simulink model "planner_contral"  (R2023b)
settings: Solver=FixedStepAuto  StartTime=0  StopTime=inf  FixedStep=0.001  RelTol=1e-3
undefined symbols (not defined in the file): aubr, c_factor, cf, cr, iniObsHeading1, iniObsHeading2, iniObsPos1, iniObsPos2, KD_PID_distance, KD_PID_speed, KI_PID_distance, KI_PID_speed, KP_PID_distance, KP_PID_speed, la, lb, LQR_K1, LQR_K2, LQR_K3, LQR_K4, m, rack_displacement, refInfo_obs1, refInfo_obs2, right_wheel_ground, rightWaypoints, tablebr, vubr, vx_break_point
libraries: Solver_SF x1
(part 5 of 8)

== matlab function planner_contral/decision_planning/EMplanner/generate convex space_base ==
  data: dp_speed_s input; s_lb output; dp_speed_t input; path_index2s input; static_obs_s_lb input; static_obs_s_ub input; static_obs_t_lb input; static_obs_t_ub input; dynamic_obs_s_lb input; dynamic_obs_s_ub input; dynaimc_obs_t_lb input; dynaimc_obs_t_ub input; s_ub output; s_dot_lb output; s_dot_ub output; trajectory_kappa_init input; max_lateral_accel input; static_s_ub output; static_s_lb output
function [s_lb,s_ub,s_dot_lb,s_dot_ub, static_s_ub,static_s_lb] = fcn(dp_speed_s,dp_speed_t,path_index2s,static_obs_s_lb,static_obs_s_ub,static_obs_t_lb,static_obs_t_ub,...
   dynamic_obs_s_lb,dynamic_obs_s_ub,dynaimc_obs_t_lb,dynaimc_obs_t_ub,trajectory_kappa_init,max_lateral_accel)
%generate convex space_base 该函数将计算出s,s_dot的上下界，开辟凸空间供二次规划使用
% dp_speed_s t 最多有16个，输出初始化n = 16
n = 16;
static_s_lb = ones(n,1)*-inf;
static_s_ub = ones(n,1)*inf;
dynamic_s_lb = ones(n,1)*-inf;
dynamic_s_ub = ones(n,1)*inf;
s_lb=ones(n,1)*-inf;
s_ub=ones(n,1)*inf;
s_dot_lb = ones(n,1)*-inf;
s_dot_ub = ones(n,1)*inf;
path_index2s_end_index = length(path_index2s);
dp_speed_end_index = length(dp_speed_s);

% path_index2s也是有缓冲的，找到有效的path_index2s的末尾的位置，赋值给path_index2s_end_index
for k = 2:length(path_index2s)
    if path_index2s(k) == 0 && path_index2s(k-1) ~= 0
        path_index2s_end_index = k - 1;
        break;
    end
    path_index2s_end_index = k;
end
% 找到dp_speed_s中有效的位置，赋值给dp_speed_end_index
for k = 1:length(dp_speed_s)
    if isnan(dp_speed_s(k))
        dp_speed_end_index = k - 1;
        break;
    end
end

for i = 1:n
    % 该循环将施加车辆动力学约束
    if isnan(dp_speed_s(i))
        break;
    end
    cur_s = dp_speed_s(i);
    % 通过插值的方式找到cur_s 所对应的曲率
    cur_kappa = interp1(path_index2s(1:path_index2s_end_index),trajectory_kappa_init(1:path_index2s_end_index),cur_s);
    % a = v^2 * k => v^2 = a/k 注意除0保护
    max_speed =  sqrt(max_lateral_accel / (abs(cur_kappa) + 1e-10));
    min_speed = 0;
    s_dot_lb(i) = min_speed;
    s_dot_ub(i) = max_speed;    
end



for i = 1:length(static_obs_s_lb)
    if isinf(static_obs_s_lb(i))
        continue;
    end
    % 取s t 直线的中点，作为obs_s obs_t 的坐标 
    static_obs_t = (static_obs_t_lb(i) + static_obs_t_ub(i)) / 2;
    static_obs_s = (static_obs_s_lb(i) + static_obs_s_ub(i)) / 2;
    % 插值找到当t = obs_t时，dp_speed_s 的值
    dp_s = interp1([0;dp_speed_t(1:dp_speed_end_index)],[0;dp_speed_s(1:dp_speed_end_index)],static_obs_t );
    if isnan(dp_s)
        continue;
    end
    [letf_index,right_index]=getTBoundindex(static_obs_t,dp_speed_t,dp_speed_end_index);
    if letf_index==0
        continue
    end
    if static_obs_s > dp_s
        % 决策为减速避让
        for m = letf_index:right_index
            % 在t_lb_index:t_ub_index的区间上 s的上界不可以超过障碍物st斜直线
            static_s_ub(m) = min(static_s_ub(m),static_obs_s_lb(i) -1.2);
        end
    else 
        % 决策为加速超车
        for  m = letf_index:right_index
             % 在t_lb_index:t_ub_index的区间上 s的下界不能小于障碍物st斜直线
            static_s_lb(m) = max(static_s_lb(m),static_obs_s_ub(i)+1.2 );
        end
    end

end
  
%计算动态障碍物上下凸空间边界
for i = 1:length(dynamic_obs_s_lb)
    if  isinf(dynamic_obs_s_lb(i))
        continue;
    end
    % 取s t 直线的中点，作为obs_s obs_t 的坐标 
    dynamic_obs_t = (dynaimc_obs_t_lb(i) + dynaimc_obs_t_ub(i)) / 2;
    dynamic_obs_s = (dynamic_obs_s_lb(i) + dynamic_obs_s_ub(i)) / 2;
    % 插值找到当t = obs_t时，dp_speed_s 的值
    dp_s = interp1([0;dp_speed_t(1:dp_speed_end_index)],[0;dp_speed_s(1:dp_speed_end_index)],dynamic_obs_t);
    if isnan(dp_s)
        continue;
    end
    [letf_index,right_index]=getTBoundindex(dynamic_obs_t,dp_speed_t,dp_speed_end_index);
    if letf_index==0
        continue
    end
    if dynamic_obs_s> dp_s
        % 决策为减速避让
        for m = letf_index:right_index
            % 在t_lb_index:t_ub_index的区间上 s的上界不可以超过障碍物st斜直线
            dynamic_s_ub(m) = min(dynamic_s_ub(m),dynamic_obs_s_lb(i) -1.2);
        end
    else 
        % 决策为加速超车
        for  m = letf_index:right_index
             % 在t_lb_index:t_ub_index的区间上 s的下界不能小于障碍物st斜直线
            dynamic_s_lb(m) = max(dynamic_s_lb(m) +1.2,dynamic_obs_s_ub(i));
        end
    end

end
%开始做决策，判断凸空间
 for k=1:n
     if isnan(dp_speed_s(k))
        break;
     end
     %该点没有动态障碍物点以及静态障碍物点
     if  isinf(static_s_lb(k))&& isinf(dynamic_s_lb(k))&&isinf(static_s_ub(k))&& isinf(dynamic_s_ub(k))
         continue
     end
     %针对曲线在静态障碍物上方
     if ~isinf(static_s_lb(k))&& isinf(dynamic_s_lb(k))&&isinf(static_s_ub(k))&& isinf(dynamic_s_ub(k))
         s_lb(k)=static_s_lb(k);
         s_ub(k)=static_s_ub(k);
       
     end
     %曲线在静态障碍物下方
     if isinf(static_s_lb(k))&& isinf(dynamic_s_lb(k))&&~isinf(static_s_ub(k))&& isinf(dynamic_s_ub(k))
         s_lb(k)=static_s_lb(k);
         s_ub(k)=static_s_ub(k);
        
     end
     %曲线在动态障碍物上方
     if isinf(static_s_lb(k))&& ~isinf(dynamic_s_lb(k))&&isinf(static_s_ub(k))&& isinf(dynamic_s_ub(k))
         s_lb(k)=dynamic_s_lb(k);
         s_ub(k)=dynamic_s_ub(k);
       
     end
     %曲线在动态障碍物下方
     if isinf(static_s_lb(k))&& isinf(dynamic_s_lb(k))&&isinf(static_s_ub(k))&& ~isinf(dynamic_s_ub(k))
         s_lb(k)=dynamic_s_lb(k);
         s_ub(k)=dynamic_s_ub(k);
        
     end
     %
     if ~isnan(static_s_ub(k))&&~isnan(dynamic_s_lb(k))
         s_lb(k)=dynamic_s_lb(k);
         s_ub(k)=static_s_ub(k);
     end
     if ~isnan(static_s_lb(k))&&~isnan(dynamic_s_ub(k))
         s_lb(k)=static_s_lb(k);
         s_ub(k)=dynamic_s_ub(k);
     end
     %
     if ~isnan(static_s_ub(k))&&~isnan(dynamic_s_ub(k))
          if dynamic_s_ub(k)>static_s_ub(k)
            s_ub(k)=static_s_ub(k);
          else
            s_ub(k)=dynamic_s_ub(k);
          end
     end
     %
     if ~isnan(static_s_lb(k))&&~isnan(dynamic_s_lb(k))
          if dynamic_s_lb(k)>static_s_lb(k)
            s_lb(k)=dynamic_s_lb(k);
          else
            s_lb(k)=static_s_lb(k);
          end
     end




end

end     

%该函数是为了获取当前t所对应的轨迹索引
function [left,right]=getTBoundindex(obs_t,dp_speed_t_,dp_speed_end_index_)
  %初始化参数
  left=0;
  right=0;
  %遍历dp_speed_t,找到当前obs_t_lb,obs_t_ub处于dp_speed_t的位置范围

  %判断索引位置
  for j=1:length(dp_speed_t_)
      %获取障碍物的t索引范围
      if dp_speed_t_(1)>obs_t           %说明障碍物当前时刻没有对应的索引值
          break;
      end
      if dp_speed_t_(j)< obs_t && dp_speed_t_(j + 1) > obs_t
          left=max(1,j);
          right=min(j+1,dp_speed_end_index_);
          break; 
      end
      if dp_speed_t_(j)== obs_t
          left=max(1,j);
          right=min(j,dp_speed_end_index_);
      end

  end

end

== matlab function planner_contral/decision_planning/EMplanner/obs/1 ==
  data: dynamic_obs_x_set_gcs input; dynamic_obs_y_set_gcs input; dynamic_obs_heading_set_gcs input; dynamic_obs_velocity_set_gcs input; dynamic_obs1_x_pre output; dynamic_obs1_y_pre output; dynamic_obs1_vx_set output; dynamic_obs1_vy_set output; pre_obs1 input
function [dynamic_obs1_x_pre,dynamic_obs1_y_pre,dynamic_obs1_vx_set,dynamic_obs1_vy_set ]...
    = fcn(dynamic_obs_x_set_gcs,dynamic_obs_y_set_gcs,dynamic_obs_heading_set_gcs,dynamic_obs_velocity_set_gcs,pre_obs1)

%该函数将分类静态障碍物和动态障碍物
%输出初始化
n = 32;

dynamic_obs1_x_pre = ones(n,1)*nan;
dynamic_obs1_y_pre = ones(n,1)*nan;
dynamic_obs1_vx_set = ones(n,1)*nan;
dynamic_obs1_vy_set = ones(n,1)*nan;
dynamic_obs1_heading_set = ones(n,1)*nan;
% dynamic_obs2_x_pre = ones(n,1)*nan;
% dynamic_obs2_y_pre = ones(n,1)*nan;
% dynamic_obs2_vx_set = ones(n,1)*nan;
% dynamic_obs2_vy_set = ones(n,1)*nan;
pre_tra_obs1_x=pre_obs1(:,1)';
pre_tra_obs1_y=pre_obs1(:,2)';
% pre_tra_obs2_x=pre_obs1(:,1)';
% pre_tra_obs2_y=pre_obs1(:,2)';
count_dynamic = 1;
for i = 1:length(dynamic_obs_x_set_gcs)
    if ~isnan(dynamic_obs_x_set_gcs(i))
        if i==1
        dynamic_obs1_x_pre(1) = dynamic_obs_x_set_gcs(i);
        dynamic_obs1_y_pre(1) =dynamic_obs_y_set_gcs(i);
            dynamic_obs1_vx_set(1) =dynamic_obs_velocity_set_gcs(i)*cos(dynamic_obs_heading_set_gcs(i));
            dynamic_obs1_vy_set(1) = dynamic_obs_velocity_set_gcs(i)*sin(dynamic_obs_heading_set_gcs(i));

         for j=1:length(pre_tra_obs1_x(1,:))
              %交换位置
            dynamic_obs1_x_pre(j+1) =pre_tra_obs1_x(1,j);
            dynamic_obs1_y_pre(j+1) =pre_tra_obs1_y(1,j);
            dynamic_obs1_vx_set(j+1) =dynamic_obs_velocity_set_gcs(i)*cos(dynamic_obs_heading_set_gcs(i));
            dynamic_obs1_vy_set(j+1) = dynamic_obs_velocity_set_gcs(i)*sin(dynamic_obs_heading_set_gcs(i));

         end
      for z=1:length(dynamic_obs1_x_pre)-1
          if dynamic_obs1_x_pre(z+1)<dynamic_obs1_x_pre(z)
              temp_x=dynamic_obs1_x_pre(z+1);
              temp_y=dynamic_obs1_y_pre(z+1);
              dynamic_obs1_x_pre(z+1)=dynamic_obs1_x_pre(z);
              dynamic_obs1_y_pre(z+1)=dynamic_obs1_y_pre(z);
              dynamic_obs1_x_pre(z)=temp_x;
              dynamic_obs1_y_pre(z)=temp_y;
          else
              break
          end
      end
 
 

      end



        %在此处增密路径变为80个点
         

           %计算动态障碍物航向角
%           [path_heading_,path_kappa_] = fcn(path_x,path_y)


        end

%         if i==2
%         dynamic_obs2_x_pre(1) = obs_x_set_gcs(i);
%         dynamic_obs2_y_pre(1) = obs_y_set_gcs(i);
%         for j=1:length(pre_tra_obs2_x(1,:))
%             dynamic_obs2_x_pre(j+1) =pre_tra_obs2_x(1,j);
%             dynamic_obs2_y_pre(j+1) =pre_tra_obs2_y(1,j);
% 
%         end 
%             dynamic_obs2_vx_set(1) = obs_velocity_set_gcs(i)*cos(obs_heading_set_gcs(i));
%             dynamic_obs2_vy_set(1) = obs_velocity_set_gcs(i)*sin(obs_heading_set_gcs(i));
%         end
%             
      count_dynamic = count_dynamic + 1;    
     end
% end

% function[tra_x,tra_y]=Den(tra_x_init,tra_y_init)
% %定义增密数组长度
% n=80;
% tra_x=ones(n,1);
% tra_y=ones(n,1);
% 
% 
% 
% 
% end
% 
% 
% 
% 
% function [path_heading,path_kappa] = fcn(path_x,path_y)
% %该函数将计算path的切线方向与x轴的夹角和曲率
% %输入：path_x,y路径坐标
% %输出：path heading kappa 路径的heading和曲率
% %原理 heading = arctan(dy/dx);
% %     kappa = dheading/ds;
% %     ds = (dx^2 + dy^2)^0.5
% 
% %注意，角度的多值性会带来很大的麻烦，需要慎重处理
% %例，x 与 x + 2pi往往代表同一个角度，这种多值性在计算曲率会带来麻烦
% %比如 原本是(0.1 - (-0.1))/ds，但如果计算出的-0.1多了一个2pi
% %kappa就等于(0.1 - (-0.1 + 2*pi))/ds，曲率会变得非常大
% %还有若采用中点欧拉法计算heading时，(即使用(y2 - y1)/(x2 - x1)的反正切计算一个角度 ，用(y1 - y0)/(x1
% %-x0)的反正切又计算一个角度，然后加起来除以2),如果精确值是 (a1 + a2)/2,但最终计算的结果可能是(a1 + a2 + 2pi)/2
% % 还有 tan(x) = tan(x + pi) 所以arctan(tan(x))可能等于x，也可能等于x + pi
% % 角度的处理非常麻烦，而且角度处理不当往往是许多奇怪错误的源头
% 
% dx = diff(path_x);
% dy = diff(path_y);
% %用中点欧拉法要比向前欧拉法向后欧拉法更精确，但是也可能计算出的结果比精确值多一个pi
% %在这里对dx,dy做中点欧拉法，使用四象限反正切计算角度
% dx_pre = [dx(1);dx];
% dx_after = [dx;dx(end)];
% dx_final = (dx_pre + dx_after)/2;
% 
% dy_pre = [dy(1);dy];
% dy_after = [dy;dy(end)];
% dy_final = (dy_pre + dy_after)/2;
% 
% ds_final = sqrt(dx_final.^2 + dy_final.^2);
% path_heading = atan2(dy_final,dx_final);
% 
% dheading = diff(path_heading);
% dheading_pre = [dheading(1);dheading];
% dheading_after = [dheading;dheading(end)];
% dheading_final = (dheading_pre + dheading_after) / 2;
% %为了防止dheading出现多一个2pi的错误，假设真实的dheading较小，用sin(dheading)近似dheading
% path_kappa = sin(dheading_final) ./ ds_final;
% end

== matlab function planner_contral/decision_planning/EMplanner/spee planning with quadratic programming (qp)_base ==
  data: plan_start_s_dot input; qp_s_init output; plan_start_s_dot2 input; dp_speed_s input; dp_speed_t input; s_lb input; s_ub input; s_dot_lb input; s_dot_ub input; qp_s_dot_init output; qp_s_dot2_init output; relative_time_init output; w_cost_s_dot2 input; w_cost_v_ref input; w_cost_jerk input; w_ref_s input; speed_reference input
function [qp_s_init,qp_s_dot_init,qp_s_dot2_init,relative_time_init] = fcn(plan_start_s_dot,...
    plan_start_s_dot2,dp_speed_s,dp_speed_t,s_lb,s_ub,s_dot_lb,s_dot_ub,w_cost_s_dot2,w_cost_v_ref,w_cost_jerk,w_ref_s,speed_reference)
%速度二次规划
% 输入：规划起点plan_start_s_dot,plan_start_s_dot2
%       动态规划结果dp_speed_s,dp_speed_t
%       凸空间约束 s_lb,s_ub,s_dot_lb,s_dot_ub
%       加速度代价权重，推荐速度代价权重，jerk代价权重w_cost_s_dot2,w_cost_v_ref,w_cost_jerk
%       参考速度speed_reference
% 输出：速度曲线qp_s_init,qp_s_dot_init,qp_s_dot2_init,relative_time_init
coder.extrinsic("quadprog")
% 由于dp的结果未必是16，该算法将计算dp_speed_end到底是多少
dp_speed_end = 16;
for i = 1:length(dp_speed_s)
    
    if isnan(dp_speed_s(i))
        dp_speed_end = i - 1;
        break;
    end
end
% 由于dp_speed_end实际上是不确定的，但是输出要求必须是确定长度的值，因此
% 输出初始化选择dp_speed_end的最大值 + 规划起点作为输出初始化的规模
n = 17;

qp_s_init = ones(n,1) * nan;
qp_s_dot_init = ones(n,1) * nan;
qp_s_dot2_init = ones(n,1) * nan;
relative_time_init = ones(n,1) * nan;
s_end = dp_speed_s(dp_speed_end);
% 此时dp_speed_end表示真正有效的dp_speed_t的元素个数，取出dp_speed_t有效的最后一个元素作为规划的时间终点
% 记为recommend_T
recommend_T = dp_speed_t(dp_speed_end);
% qp的规模应该是dp的有效元素的个数 + 规划起点
qp_size = dp_speed_end + 1;
% 连续性约束矩阵初始化，这里的等式约束应该是 Aeq'*X == beq 有转置
Aeq = zeros(3*qp_size,2*qp_size - 2);
beq = zeros(2*qp_size - 2,1);
% 不等式约束初始化
lb = ones(3*qp_size,1);
ub = lb;
% 计算采样间隔时间dt,连续性约束
dt = recommend_T/dp_speed_end;
A_sub =[1,0;
        dt,1;
        (1/3)*dt^2,(1/2)*dt;
        -1,0;
        0,-1;
        (1/6)*dt^2,dt/2];
for i = 1:qp_size - 1
    Aeq(3*i-2:3*i+3,2*i-1:2*i) = A_sub;
end
% 这里初始化不允许倒车约束，也就是 s(i) - s(i+1) <= 0
A = zeros(qp_size-1,3*qp_size);
b = zeros(qp_size-1,1);
for i = 1:qp_size-1
    A(i,3*i - 2) = 1;
    A(i,3*i + 1) = -1;
end
% 由于生成的凸空间约束s_lb s_ub不带起点，所以lb(i) = s_lb(i-1) 以此类推
% 允许最小加速度为-6 最大加速度为4(基于车辆动力学)
for i = 2:qp_size
   lb(3*i - 2) = s_lb(i-1);
   lb(3*i - 1) = s_dot_lb(i-1);
   lb(3*i) = -6;
   ub(3*i - 2) = s_ub(i-1);
   ub(3*i - 1) = s_dot_ub(i-1);
   ub(3*i) = 4;
end
% 起点约束
lb(1) = 0;
lb(2) = plan_start_s_dot;
lb(3) = plan_start_s_dot2;
ub(1) = lb(1);
ub(2) = lb(2);
ub(3) = lb(3);
% 加速度代价 jerk代价 以及推荐速度代价
A_s_dot2 = zeros(3*qp_size,3*qp_size);
A_jerk = zeros(3*qp_size,qp_size - 1);
A_ref = zeros(3*qp_size,3*qp_size);
A_ref_s = zeros(3*qp_size,3*qp_size);
A4_sub =[0;0;1;0;0;-1];
for i = 1:qp_size
    A_s_dot2(3*i,3*i) = 1;
    A_ref(3*i-1,3*i-1) = 1;
    A_ref_s(3*i-2,3*i-2)=1;
end
for i = 1:qp_size - 1   
   A_jerk(3*i-2:3*i+3,i:i) = A4_sub;
end
% 生成H f
H = w_cost_s_dot2 * (A_s_dot2 * A_s_dot2') + w_cost_jerk * (A_jerk * A_jerk') + w_cost_v_ref * (A_ref * A_ref')+w_ref_s*(A_ref_s * A_ref_s');
H = 2*H;
f = zeros(3*qp_size,1);
for i = 1:qp_size
    f(3*i-1) =  - 2 * w_cost_v_ref * speed_reference;  %这里应该晖多加一个代价
   
end
for i=1:dp_speed_end
      f(3*i-2) =  - 2 * w_ref_s * dp_speed_s(i);  %这里应该晖多加一个代价
end

% 计算二次规划
X = quadprog(H,f,A,b,Aeq',beq,lb,ub);
% 将结果输出
for i = 1:qp_size
   qp_s_init(i) = X(3*i - 2);
   qp_s_dot_init(i) = X(3*i - 1);
   qp_s_dot2_init(i) = X(3*i);
   relative_time_init(i) = (i - 1)*dt;
end

== matlab function planner_contral/decision_planning/EMplanner/spee planning with quadratic programming (qp)_1 ==
  data: plan_start_s_dot input; qp_s_init output; plan_start_s_dot2 input; dp_speed_s input; dp_speed_t input; s_lb input; s_ub input; s_dot_lb input; s_dot_ub input; qp_s_dot_init output; qp_s_dot2_init output; relative_time_init output; w_cost_s_dot2 input; w_cost_v_ref input; w_cost_jerk input; w_ref_s input; speed_reference input
function [qp_s_init,qp_s_dot_init,qp_s_dot2_init,relative_time_init] = fcn(plan_start_s_dot,...
    plan_start_s_dot2,dp_speed_s,dp_speed_t,s_lb,s_ub,s_dot_lb,s_dot_ub,w_cost_s_dot2,w_cost_v_ref,w_cost_jerk,w_ref_s,speed_reference)
%速度二次规划
% 输入：规划起点plan_start_s_dot,plan_start_s_dot2
%       动态规划结果dp_speed_s,dp_speed_t
%       凸空间约束 s_lb,s_ub,s_dot_lb,s_dot_ub
%       加速度代价权重，推荐速度代价权重，jerk代价权重w_cost_s_dot2,w_cost_v_ref,w_cost_jerk
%       参考速度speed_reference
% 输出：速度曲线qp_s_init,qp_s_dot_init,qp_s_dot2_init,relative_time_init
coder.extrinsic("quadprog")
% 由于dp的结果未必是16，该算法将计算dp_speed_end到底是多少
dp_speed_end = 16;
for i = 1:length(dp_speed_s)
    
    if isnan(dp_speed_s(i))
        dp_speed_end = i - 1;
        break;
    end
end
% 由于dp_speed_end实际上是不确定的，但是输出要求必须是确定长度的值，因此
% 输出初始化选择dp_speed_end的最大值 + 规划起点作为输出初始化的规模
n = 17;

qp_s_init = ones(n,1) * nan;
qp_s_dot_init = ones(n,1) * nan;
qp_s_dot2_init = ones(n,1) * nan;
relative_time_init = ones(n,1) * nan;
s_end = dp_speed_s(dp_speed_end);
% 此时dp_speed_end表示真正有效的dp_speed_t的元素个数，取出dp_speed_t有效的最后一个元素作为规划的时间终点
% 记为recommend_T
recommend_T = dp_speed_t(dp_speed_end);
% qp的规模应该是dp的有效元素的个数 + 规划起点
qp_size = dp_speed_end + 1;
% 连续性约束矩阵初始化，这里的等式约束应该是 Aeq'*X == beq 有转置
Aeq = zeros(3*qp_size,2*qp_size - 2);
beq = zeros(2*qp_size - 2,1);
% 不等式约束初始化
lb = ones(3*qp_size,1);
ub = lb;
% 计算采样间隔时间dt,连续性约束
dt = recommend_T/dp_speed_end;
A_sub =[1,0;
        dt,1;
        (1/3)*dt^2,(1/2)*dt;
        -1,0;
        0,-1;
        (1/6)*dt^2,dt/2];
for i = 1:qp_size - 1
    Aeq(3*i-2:3*i+3,2*i-1:2*i) = A_sub;
end
% 这里初始化不允许倒车约束，也就是 s(i) - s(i+1) <= 0
A = zeros(qp_size-1,3*qp_size);
b = zeros(qp_size-1,1);
for i = 1:qp_size-1
    A(i,3*i - 2) = 1;
    A(i,3*i + 1) = -1;
end
% 由于生成的凸空间约束s_lb s_ub不带起点，所以lb(i) = s_lb(i-1) 以此类推
% 允许最小加速度为-6 最大加速度为4(基于车辆动力学)
for i = 2:qp_size
   lb(3*i - 2) = s_lb(i-1);
   lb(3*i - 1) = s_dot_lb(i-1);
   lb(3*i) = -6;
   ub(3*i - 2) = s_ub(i-1);
   ub(3*i - 1) = s_dot_ub(i-1);
   ub(3*i) = 4;
end
% 起点约束
lb(1) = 0;
lb(2) = plan_start_s_dot;
lb(3) = plan_start_s_dot2;
ub(1) = lb(1);
ub(2) = lb(2);
ub(3) = lb(3);
% 加速度代价 jerk代价 以及推荐速度代价
A_s_dot2 = zeros(3*qp_size,3*qp_size);
A_jerk = zeros(3*qp_size,qp_size - 1);
A_ref = zeros(3*qp_size,3*qp_size);
A_ref_s = zeros(3*qp_size,3*qp_size);
A4_sub =[0;0;1;0;0;-1];
for i = 1:qp_size
    A_s_dot2(3*i,3*i) = 1;
    A_ref(3*i-1,3*i-1) = 1;
    A_ref_s(3*i-2,3*i-2)=1;
end
for i = 1:qp_size - 1   
   A_jerk(3*i-2:3*i+3,i:i) = A4_sub;
end
% 生成H f
H = w_cost_s_dot2 * (A_s_dot2 * A_s_dot2') + w_cost_jerk * (A_jerk * A_jerk') + w_cost_v_ref * (A_ref * A_ref')+w_ref_s*(A_ref_s * A_ref_s');
H = 2*H;
f = zeros(3*qp_size,1);
for i = 1:qp_size
    f(3*i-1) =  - 2 * w_cost_v_ref * speed_reference;  %这里应该晖多加一个代价
   
end
for i=1:dp_speed_end
      f(3*i-2) =  - 2 * w_ref_s * dp_speed_s(i);  %这里应该晖多加一个代价
end

% 计算二次规划
X = quadprog(H,f,A,b,Aeq',beq,lb,ub);
% 将结果输出
for i = 1:qp_size
   qp_s_init(i) = X(3*i - 2);
   qp_s_dot_init(i) = X(3*i - 1);
   qp_s_dot2_init(i) = X(3*i);
   relative_time_init(i) = (i - 1)*dt;
end

== matlab function planner_contral/decision_planning/EMplanner/generate convex space_new1 ==
  data: dp_speed_s input; s_lb output; dp_speed_t input; path_index2s input; static_obs_s_lb input; static_obs_s_ub input; static_obs_t_lb input; static_obs_t_ub input; dynamic_obs_s_lb input; dynamic_obs_s_ub input; dynamic_obs_t_lb input; dynamic_obs_t_ub input; s_ub output; s_dot_lb output; s_dot_ub output; trajectory_kappa_init input; max_lateral_accel input; static_s_ub output; static_s_lb output
%% 基于 DP 粗速度解的连续双边 ST 可行域重构
% 作用：
% 1. 根据 DP 粗解生成 QP 的 s 方向双边约束
% 2. 根据静态/动态障碍物 ST 边界裁剪可行域
% 3. 修复障碍物边界退化、可行域过窄、相邻点不连续等问题
% 4. 输出 QP 速度规划需要的 s_lb/s_ub/s_dot_lb/s_dot_ub

% ============================================================
% 基本参数
% ============================================================
function [s_lb,s_ub,s_dot_lb,s_dot_ub, static_s_ub,static_s_lb] = fcn( ...
    dp_speed_s,dp_speed_t,path_index2s, ...
    static_obs_s_lb,static_obs_s_ub,static_obs_t_lb,static_obs_t_ub, ...
    dynamic_obs_s_lb,dynamic_obs_s_ub,dynamic_obs_t_lb,dynamic_obs_t_ub, ...
    trajectory_kappa_init,max_lateral_accel)

n = 16;

safe_margin = 1.0;        % 障碍物纵向安全距离
back_margin = 10.0;       % DP 曲线后方保留距离
front_margin = 14.0;      % DP 曲线前方保留距离
min_width = 6.0;          % QP 可行域最小宽度
s_floor = 0.0;            % 局部 s 下界
default_speed_ub = 30.0;  % 默认速度上界

acc_min = -6.0;           % 最小加速度
acc_max = 4.0;            % 最大加速度

% QP 速度规划采样点：0.5s 到 8s
t_qp = (0.5:0.5:8.0)';

% ST 图时间采样点：0s 到 8s，间隔 0.1s
t_st = (0:0.1:8.0)';

% ============================================================
% 输出初始化
% ============================================================
s_lb = zeros(n,1);
s_ub = zeros(n,1);

static_s_lb = ones(n,1) * -inf;
static_s_ub = ones(n,1) * inf;

s_dot_lb = zeros(n,1);
s_dot_ub = ones(n,1) * default_speed_ub;

% ============================================================
% 整理 DP 粗速度解
% ============================================================
valid_dp = isfinite(dp_speed_s) & isfinite(dp_speed_t);
dp_s_valid = dp_speed_s(valid_dp);
dp_t_valid = dp_speed_t(valid_dp);

if isempty(dp_s_valid)
    % 如果 DP 没有有效解，则给一个保守但不崩溃的默认可行域
    for i = 1:n
        s_lb(i) = s_floor;
        s_ub(i) = front_margin + 5.0 * i;
    end

    % s_dot_ub = calcSpeedUpperBound(trajectory_kappa_init, max_lateral_accel, ...
    %                                default_speed_ub, n);
    s_dot_ub = ones(n,1) * default_speed_ub;
    return;
end

% 保证 DP 时间单调
[dp_t_valid, order] = sort(dp_t_valid);
dp_s_valid = dp_s_valid(order);

% 去掉重复时间点，避免 interp1 出错
[dp_t_valid, uniqueIdx] = unique(dp_t_valid, 'stable');
dp_s_valid = dp_s_valid(uniqueIdx);

% 将 DP 粗解插值到 QP 采样点
s_dp_qp = interpHold(dp_t_valid, dp_s_valid, t_qp);

% ============================================================
% 以 DP 曲线为中心，初始化双边可行域
% ============================================================
for i = 1:n
    s_lb(i) = max(s_floor, s_dp_qp(i) - back_margin);
    s_ub(i) = s_dp_qp(i) + front_margin;
end

% ============================================================
% 静态障碍物约束裁剪
% ============================================================
for i = 1:n
    [obs_lb, obs_ub, has_obs] = getObstacleBoundAtTime( ...
        t_qp(i), t_st, static_obs_s_lb, static_obs_s_ub);

    if has_obs
        static_s_lb(i) = obs_lb;
        static_s_ub(i) = obs_ub;

        [s_lb(i), s_ub(i)] = clipCorridorByObstacle( ...
            s_lb(i), s_ub(i), s_dp_qp(i), obs_lb, obs_ub, safe_margin);
    end
end

% ============================================================
% 动态障碍物约束裁剪
% ============================================================
for i = 1:n
    [obs_lb, obs_ub, has_obs] = getObstacleBoundAtTime( ...
        t_qp(i), t_st, dynamic_obs_s_lb, dynamic_obs_s_ub);

    if has_obs
        [s_lb(i), s_ub(i)] = clipCorridorByObstacle( ...
            s_lb(i), s_ub(i), s_dp_qp(i), obs_lb, obs_ub, safe_margin);
    end
end

% ============================================================
% 基础可行性修复
% ============================================================
for i = 1:n
    if ~isfinite(s_lb(i))
        s_lb(i) = s_floor;
    end

    if ~isfinite(s_ub(i))
        s_ub(i) = s_dp_qp(i) + front_margin;
    end

    s_lb(i) = max(s_lb(i), s_floor);

    if s_ub(i) <= s_lb(i) + min_width
        if s_dp_qp(i) >= s_lb(i) && s_dp_qp(i) <= s_ub(i)
            s_lb(i) = max(s_floor, s_dp_qp(i) - 0.5 * min_width);
            s_ub(i) = s_lb(i) + min_width;
        elseif s_dp_qp(i) < s_lb(i)
            s_ub(i) = s_lb(i) + min_width;
        else
            s_lb(i) = max(s_floor, s_ub(i) - min_width);
        end
    end
end

% ============================================================
% 动力学可达性修复
% 说明：
% 当前函数接口没有 plan_start_s_dot 和 plan_start_s_dot2，
% 所以这里用 DP 曲线估计一个可达参考，再用它修复可行域。
% ============================================================
[s_lb, s_ub] = repairReachableCorridor( ...
    s_lb, s_ub, s_dp_qp, acc_min, acc_max, min_width, s_floor, front_margin);

% ============================================================
% 最终单调性和宽度修复
% ============================================================
for i = 2:n
    if s_lb(i) < s_lb(i-1)
        s_lb(i) = s_lb(i-1);
    end

    if s_ub(i) < s_ub(i-1)
        s_ub(i) = s_ub(i-1);
    end

    if s_ub(i) <= s_lb(i) + min_width
        s_ub(i) = s_lb(i) + min_width;
    end
end

% ============================================================
% 速度上下界
% ============================================================
s_dot_lb = zeros(n,1);
% s_dot_ub = calcSpeedUpperBound(trajectory_kappa_init, max_lateral_accel, ...
%                                default_speed_ub, n);
s_dot_ub = ones(n,1) * default_speed_ub;
end
%%
% 根据 DP 粗解选择从障碍物前方还是后方通过
% s_dp < obs_lb：DP 在障碍物后方，约束上界
% s_dp > obs_ub：DP 在障碍物前方，约束下界
% s_dp 在障碍物内部：选择修正量较小的一侧
function [new_lb, new_ub] = clipCorridorByObstacle( ...
    cur_lb, cur_ub, s_dp, obs_lb, obs_ub, safe_margin)

new_lb = cur_lb;
new_ub = cur_ub;

if ~isfinite(obs_lb) || ~isfinite(obs_ub)
    return;
end

if obs_ub < obs_lb
    temp = obs_lb;
    obs_lb = obs_ub;
    obs_ub = temp;
end

if s_dp < obs_lb
    new_ub = min(new_ub, obs_lb - safe_margin);
elseif s_dp > obs_ub
    new_lb = max(new_lb, obs_ub + safe_margin);
else
    dist_to_lb = abs(s_dp - obs_lb);
    dist_to_ub = abs(s_dp - obs_ub);

    if dist_to_lb <= dist_to_ub
        new_ub = min(new_ub, obs_lb - safe_margin);
    else
        new_lb = max(new_lb, obs_ub + safe_margin);
    end
end

end

%%
% 从 ST 图中读取指定时间 t 对应的障碍物 s 边界
% 同时修复 lb == ub 的退化情况
function [obs_lb, obs_ub, has_obs] = getObstacleBoundAtTime(t, t_grid, obs_lb_set, obs_ub_set)

% 从 ST 图中读取指定时间 t 对应的障碍物 s 边界
% 支持 0 个、1 个、多个有效 ST 点
% 如果只有 1 个有效点，不做 interp1，直接在该点附近短时间内保持

obs_lb = inf;
obs_ub = -inf;
has_obs = false;

obs_min_width = 5.0;      % 障碍物 ST 纵向最小占用宽度
single_t_window = 0.25;   % 单点 ST 障碍物的时间保持窗口

valid = isfinite(obs_lb_set) & isfinite(obs_ub_set);

if ~any(valid)
    return;
end

t_valid = t_grid(valid);
lb_valid = obs_lb_set(valid);
ub_valid = obs_ub_set(valid);

num_valid = length(t_valid);

if num_valid == 0
    return;
end

if num_valid == 1
    % 只有一个有效 ST 点时，不能使用 interp1
    % 如果当前 QP 时间点离这个 ST 点较近，则认为障碍物有效
    if abs(t - t_valid(1)) > single_t_window
        return;
    end

    obs_lb = lb_valid(1);
    obs_ub = ub_valid(1);
else
    % 多个有效点时，使用线性插值
    if t < t_valid(1) || t > t_valid(end)
        return;
    end

    obs_lb = interp1(t_valid, lb_valid, t, 'linear');
    obs_ub = interp1(t_valid, ub_valid, t, 'linear');
end

if isfinite(obs_lb) && isfinite(obs_ub)
    if obs_ub < obs_lb
        temp = obs_lb;
        obs_lb = obs_ub;
        obs_ub = temp;
    end

    % 防止障碍物边界退化成一个点
    if obs_ub - obs_lb < obs_min_width
        obs_center = 0.5 * (obs_lb + obs_ub);
        obs_lb = obs_center - 0.5 * obs_min_width;
        obs_ub = obs_center + 0.5 * obs_min_width;
    end

    has_obs = true;
end

end


%% 线性插值，两端采用保持策略
function yq = interpHold(x, y, xq)

yq = zeros(size(xq));

if numel(x) == 1
    yq(:) = y(1);
    return;
end

for i = 1:numel(xq)
    if xq(i) <= x(1)
        yq(i) = y(1);
    elseif xq(i) >= x(end)
        yq(i) = y(end);
    else
        yq(i) = interp1(x, y, xq(i), 'linear');
    end
end

end

%% 根据 DP 曲线估计一个动力学可达参考点
% 再用该参考点修复 s_lb/s_ub，避免 QP 因动力学不可达而无解
function [s_lb, s_ub] = repairReachableCorridor( ...
    s_lb, s_ub, s_dp, acc_min, acc_max, min_width, s_floor, front_margin)

n = length(s_lb);
dt = 0.5;

s_ref = zeros(n,1);
v_ref = zeros(n,1);

s_ref(1) = s_dp(1);
v_ref(1) = max(0, s_dp(1) / dt);

for i = 2:n
    v_des = (s_dp(i) - s_ref(i-1)) / dt;

    v_low = max(0, v_ref(i-1) + acc_min * dt);
    v_high = max(v_low, v_ref(i-1) + acc_max * dt);

    v_ref(i) = min(max(v_des, v_low), v_high);
    s_ref(i) = s_ref(i-1) + v_ref(i) * dt;
end

for i = 1:n
    if ~isfinite(s_lb(i))
        s_lb(i) = s_floor;
    end

    if ~isfinite(s_ub(i))
        s_ub(i) = s_ref(i) + front_margin;
    end

    s_lb(i) = max(s_lb(i), s_floor);

    if s_ref(i) >= s_lb(i) && s_ref(i) <= s_ub(i)
        if s_ub(i) - s_lb(i) < min_width
            s_lb(i) = max(s_floor, s_ref(i) - 0.5 * min_width);
            s_ub(i) = s_lb(i) + min_width;
        end
    elseif s_ref(i) < s_lb(i)
        s_ub(i) = max(s_ub(i), s_lb(i) + min_width);
    else
        s_lb(i) = min(s_lb(i), s_ub(i) - min_width);
        s_lb(i) = max(s_lb(i), s_floor);
    end

    if s_ub(i) <= s_lb(i) + min_width
        s_ub(i) = s_lb(i) + min_width;
    end
end

end

%% 根据横向加速度限制计算速度上界
% v <= sqrt(a_lat_max / abs(kappa))
function s_dot_ub = calcSpeedUpperBound(trajectory_kappa_init, max_lateral_accel, default_speed_ub, n)

s_dot_ub = ones(n,1) * default_speed_ub;

if ~isfinite(max_lateral_accel) || max_lateral_accel <= 0
    return;
end

for i = 1:n
    if i <= length(trajectory_kappa_init)
        kappa = abs(trajectory_kappa_init(i));

        if isfinite(kappa) && kappa > 1e-6
            v_max = sqrt(max_lateral_accel / kappa);

            if isfinite(v_max)
                s_dot_ub(i) = min(default_speed_ub, v_max);
            end
        end
    end

    % 防止曲率异常导致速度上界过小
    if s_dot_ub(i) < 1.0
        s_dot_ub(i) = 1.0;
    end
end

end

== matlab function planner_contral/decision_planning/EMplanner/genrate index to s ==
  data: path_x input; index2s output; path_y input; origin_x input; origin_y input; origin_match_point_index input
function index2s  = fcn(path_x,path_y,origin_x,origin_y,origin_match_point_index)
%该函数将输出index与s的转换关系，index2s表示当path_x,path_y的离散点的编号为i时，对应的弧长为index2s(i)
%输入 path_x path_y 待转化的离散点的集合
% origin_x,y frenet原点在世界坐标系下的坐标,也就是投影点
% origin_match_point_index 原点的匹配点的编号
%apollo的轨迹拼接的s与t是针对匹配点计算的累计距离s与t，通每个点-匹配点的是S,T
% path点的个数
n = 121;
% 输出初始化
index2s = zeros(n,1);
% 首先计算以path起点为坐标原点的index2s
for i = 2:n
    index2s(i) = sqrt((path_x(i) - path_x(i-1))^2 + (path_y(i) - path_y(i-1))^2) + index2s(i-1);  %计算没一段的弧长
end
% 再计算以轨迹起点到frenet_path的坐标原点的弧长，记为s0，再用index2s - s0 就是最终的结果
% 计算s0
% s_temp 匹配点的弧长
s_temp = index2s(origin_match_point_index);   
%判断投影点在匹配点的前面还是后面
vector_match_2_origin = [origin_x;origin_y] - [path_x(origin_match_point_index);path_y(origin_match_point_index)];
vector_match_2_match_next = [path_x(origin_match_point_index + 1);path_y(origin_match_point_index + 1)] - ...
                            [path_x(origin_match_point_index);path_y(origin_match_point_index)];
if vector_match_2_origin'*vector_match_2_match_next > 0
    %投影点在匹配点的前面
    s0 = s_temp + sqrt(vector_match_2_origin'*vector_match_2_origin);   %点乘投影
else
    %投影点在匹配点的后面
    s0 = s_temp - sqrt(vector_match_2_origin'*vector_match_2_origin);
end
%移动的弧长,这段弧长说明匹配点前面的所有点都是负数，只有匹配点后面的为整数，相对s
index2s = index2s - ones(n,1)*s0;

== matlab function planner_contral/global_path_info/Separation trajectory ==
  data: global_xy input; global_x_ output; global_y_ output
function [global_x_,global_y_] = fcn(global_xy)
global_xy_=global_xy;
  n=length(global_xy_(:,1));
  global_x_=zeros(n,1);
  global_y_=zeros(n,1);

  for i=1:n
      global_x_(i,1)=global_xy_(i,1);
  end
  for j=1:n
      global_y_(j,1)=global_xy_(j,2);

  end
end

== matlab function planner_contral/decision_planning/EMplanner/Cartesian2Frenet/MATLAB Function1 ==
  data: l_set input; s_dot_set output; vx_set input; vy_set input; proj_heading_set input; proj_kappa_set input; l_dot_set output; dl_set output
function [s_dot_set,l_dot_set,dl_set] = fcn(l_set,vx_set,vy_set,proj_heading_set,proj_kappa_set)
%该函数将计算frenet坐标系下的s_dot, l_dot, dl/ds
n = 128;
% 输出初始化
s_dot_set = ones(n,1)*nan;
l_dot_set = ones(n,1)*nan;
dl_set = ones(n,1)*nan;

for i = 1 : length(l_set)
    if isnan(l_set(i))
        break;
    end
    v_h = [vx_set(i);vy_set(i)];
    n_r = [-sin(proj_heading_set(i));cos(proj_heading_set(i))];
    t_r = [cos(proj_heading_set(i));sin(proj_heading_set(i))];
    l_dot_set(i) = v_h'*n_r;
    s_dot_set(i) = v_h'*t_r/(1 - proj_kappa_set(i)*l_set(i));
    %%%向量法做cartesian与frenet的转换要更简单，但是也有缺点，向量法必须依赖速度加速度
    %l' = l_dot/s_dot 但是如果s_dot = 0 此方法就失效了
    if abs(s_dot_set(i)) < 1e-6
        dl_set(i) = 0;
    else
        dl_set(i) = l_dot_set(i)/s_dot_set(i);
    end
end

== matlab function planner_contral/decision_planning/EMplanner/Cartesian2Frenet/MATLAB Function ==
  data: x_set input; s_set output; y_set input; frenet_path_x input; frenet_path_y input; proj_x_set input; proj_y_set input; proj_heading_set input; proj_match_point_index_set input; index2s input; l_set output
function [s_set,l_set] = fcn(x_set,y_set,frenet_path_x,frenet_path_y,...
    proj_x_set,proj_y_set,proj_heading_set,proj_match_point_index_set,index2s)
    %该函数将计算世界坐标系下的x_set，y_set上的点在frenet_path下的坐标s l
    %输入 x_set,y_set 待坐标转换的点
    %     frenet_path_x,frenet_path_y   frenet坐标轴
    %     proj_x,y,heading,kappa,proj_match_point_index 待坐标转换的点的投影点的信息
    %     index2s   frenet_path的index与s的转换表

    % 由于不知道有多少个点需要做坐标转换，所以需要做缓冲
    n = 128;%最多处理128个点
    %输出初始化
    s_set = ones(n,1)*nan;
    l_set = ones(n,1)*nan;
    for i = 1:length(x_set)
        if isnan(x_set(i))
            break;
        end
        %计算s，写个子函数
        s_set(i) = CalcSFromIndex2S(index2s,frenet_path_x,frenet_path_y,proj_x_set(i),proj_y_set(i),...
            proj_match_point_index_set(i));
        n_r = [-sin(proj_heading_set(i));cos(proj_heading_set(i))];
        r_h = [x_set(i);y_set(i)];
        r_r = [proj_x_set(i);proj_y_set(i)];
        l_set(i) = (r_h - r_r)'*n_r;
    end
end

function s = CalcSFromIndex2S(index2s,path_x,path_y,proj_x,proj_y,proj_match_point_index)
  %该函数将计算当指定index2s的映射关系后，计算点proj_x,proj_y的弧长
  vector_1 = [proj_x;proj_y] - [path_x(proj_match_point_index);path_y(proj_match_point_index)];
  %这里要考虑的更全面一些，因为要考虑到proj_match_point_index有可能在path的起点或终点
  if (proj_match_point_index < length(path_x))
      vector_2 = [path_x(proj_match_point_index + 1);path_y(proj_match_point_index + 1)] - ...
          [path_x(proj_match_point_index);path_y(proj_match_point_index)];
  else
      vector_2 = [path_x(proj_match_point_index);path_y(proj_match_point_index)] - ...
          [path_x(proj_match_point_index - 1);path_y(proj_match_point_index - 1)];
  end
  
  if vector_1'*vector_2 > 0
      s = index2s(proj_match_point_index) + sqrt(vector_1'*vector_1);
  else
      s = index2s(proj_match_point_index) - sqrt(vector_1'*vector_1);
  end
  
  
end

== matlab function planner_contral/decision_planning/EMplanner/Frenet2Cartesian task ==
  data: s_set input; x_set output; l_set input; dl_set input; ddl_set input; frenet_path_x input; frenet_path_y input; frenet_path_heading input; frenet_path_kappa input; index2s input; y_set output; heading_set output; kappa_set output
function [x_set,y_set,heading_set,kappa_set] = ...
    fcn(s_set,l_set,dl_set,ddl_set,frenet_path_x,frenet_path_y,frenet_path_heading,frenet_path_kappa,index2s)
% 通用算法 frenet转cartesian
% 由于不知道有多少个(s,l)要转化成直角坐标，因此做缓冲
% 输出初始化
    x_set = ones(600,1) * nan;
    y_set = ones(600,1) * nan;
    heading_set = ones(600,1) * nan;
    kappa_set = ones(600,1) * nan;
    for i = 1:length(s_set)
        if isnan(s_set(i))
            break;
        end
        % 计算(s,l)在frenet坐标轴上的投影
        [proj_x,proj_y,proj_heading,proj_kappa] = CalcProjPoint(s_set(i),frenet_path_x,frenet_path_y,frenet_path_heading,...
    frenet_path_kappa,index2s);
        nor = [-sin(proj_heading);cos(proj_heading)];
        point = [proj_x;proj_y] + l_set(i) * nor;
        x_set(i) = point(1);
        y_set(i) = point(2);
        heading_set(i) = proj_heading + atan(dl_set(i)/(1 - proj_kappa * l_set(i)));
        % 近似认为 kappa' == 0,frenet转cartesian公式，见第一章第三节评论区的链接
        kappa_set(i) = ((ddl_set(i) + proj_kappa * dl_set(i) * tan(heading_set(i) - proj_heading)) * ...
            (cos(heading_set(i) - proj_heading)^2)/(1 - proj_kappa * l_set(i)) + proj_kappa) * ...
            cos(heading_set(i) - proj_heading)/(1 - proj_kappa * l_set(i));
         
    end

end


function [proj_x,proj_y,proj_heading,proj_kappa] = CalcProjPoint(s,frenet_path_x,frenet_path_y,frenet_path_heading,...
    frenet_path_kappa,index2s)
% 该函数将计算在frenet坐标系下，点(s,l)在frenet坐标轴的投影的直角坐标(proj_x,proj_y,proj_heading,proj_kappa)'
% 先找匹配点的编号
    match_index = 1;
    while index2s(match_index) < s
        match_index = match_index + 1;
    end
    match_point = [frenet_path_x(match_index);frenet_path_y(match_index)];
    match_point_heading = frenet_path_heading(match_index);
    match_point_kappa = frenet_path_kappa(match_index);
    ds = s - index2s(match_index);
    match_tor = [cos(match_point_heading);sin(match_point_heading)];
    proj_point = match_point + ds * match_tor;
    proj_heading = match_point_heading + ds * match_point_kappa;
    proj_kappa = match_point_kappa;
    proj_x = proj_point(1);
    proj_y = proj_point(2);   
end

== matlab function planner_contral/decision_planning/EMplanner/MATLAB Function1 ==
  data: x_set input; match_point_index_set output; y_set input; frenet_path_x input; frenet_path_y input; frenet_path_heading input; frenet_path_kappa input; proj_x_set output; proj_y_set output; proj_heading_set output; proj_kappa_set output
function [match_point_index_set,proj_x_set, proj_y_set,proj_heading_set,proj_kappa_set] = ...
    fcn(x_set,y_set,frenet_path_x,frenet_path_y,frenet_path_heading,frenet_path_kappa)
%该函数将批量计算x_set，y_set中的xy，在frenet_path下的投影的信息
%输入 x_set,y_set，待投影的点的集合
%x_set,y_set,frenet_path_x,frenet_path_y,frenet_path_heading,frenet_path_kappa
%曲线在直角坐标系下的x，y，heading，kappa
%输出：match_point_index_set 匹配点在frenet_path下的编号的集合(即从全局路径第一个点开始数，第几个点是匹配点)
%     proj_x y heading kappa 投影的x,y,heading,kappa的集合

% 由于事先不知道x_set中到底有多少个点需要投影，因此事先声明一个最大的数量的点作为缓冲
n = 128;
% 并且由于不知道投影点的个数，所以也不知道输出的个数，因此输出也要做缓冲，用nan表示不存在的点
% 输出最多输出128个
% 输出初始化
match_point_index_set = ones(n,1) * nan;
proj_x_set = ones(n,1) * nan;
proj_y_set = ones(n,1) * nan;
proj_heading_set = ones(n,1) * nan;
proj_kappa_set = ones(n,1) * nan;

% 找匹配点，需要利用上一个周期的结果作为下一个周期遍历的起点，因此需要声明两个全局变量

persistent is_first_run;
persistent pre_match_point_index_set;%bug :pre_match_point_index(i) 未必代表的是第i个障碍物的match_point_index
persistent pre_frenet_path_x;
persistent pre_frenet_path_y;
persistent pre_frenet_path_heading;
persistent pre_frenet_path_kappa;
persistent pre_x_set;
persistent pre_y_set;
%算法主函数入口

if isempty(is_first_run)
    %该if分支表示函数首次运行
    is_first_run = 0;
    pre_frenet_path_x = frenet_path_x;
    pre_frenet_path_y = frenet_path_y;
    pre_frenet_path_heading = frenet_path_heading;
    pre_frenet_path_kappa = frenet_path_kappa;
    %要记录首次运行计算的匹配点的结果供下个周期运行，先初始化
    pre_match_point_index_set = ones(n,1) * nan;
    %对x_set,y_set的点做遍历，找到他们的匹配点
    for i = 1 : length(x_set)
        if isnan(x_set(i))
            break;
        end
        %首次运行时，没有任何提示，只能从frenet path的第一个点开始找
        start_search_index = 1;
        % 声明increase_count，用于表示在遍历时distance连续增加的个数
        increase_count = 0;
        % 开始遍历
        min_distance = inf;
        for j = start_search_index : length(frenet_path_x)
            distance = (x_set(i) - frenet_path_x(j))^2 + (y_set(i) - frenet_path_y(j))^2;
            if distance < min_distance
                min_distance = distance;
                match_point_index_set(i) = j;
                increase_count = 0;
            else
                increase_count = increase_count + 1;
            end
            %如果distance连续增加50次就不要再遍历了，节省时间
            if increase_count > 50
                break;
            end
        end
        
        %如何通过匹配点计算投影点，请参见《自动驾驶控制算法第七讲》
        %或《自动驾驶决策规划算法》第一章第三节
        
        %取出匹配点的编号
        match_point_index = match_point_index_set(i);
        %取出匹配点的信息
        match_point_x = frenet_path_x(match_point_index);
        match_point_y = frenet_path_y(match_point_index);
        match_point_heading = frenet_path_heading(match_point_index);
        match_point_kappa = frenet_path_kappa(match_point_index);
        %计算匹配点的方向向量与法向量
        vector_match_point = [match_point_x;match_point_y];
        vector_match_point_direction = [cos(match_point_heading);sin(match_point_heading)];
        %声明待投影点的位矢
        vector_r = [x_set(i);y_set(i)];
        
       %通过匹配点计算投影点
       vector_d = vector_r - vector_match_point;
       ds = vector_d' * vector_match_point_direction;
       vector_proj_point = vector_match_point + ds * vector_match_point_direction;
       proj_heading = match_point_heading + match_point_kappa * ds;
       proj_kappa = match_point_kappa;
       %计算结果输出
       proj_x_set(i) = vector_proj_point(1);
       proj_y_set(i) = vector_proj_point(2);
       proj_heading_set(i) = proj_heading;
       proj_kappa_set(i) = proj_kappa;
    end
    %匹配点的计算结果保存，供下一个周期使用
    pre_match_point_index_set = match_point_index_set;
    pre_x_set = x_set;
    pre_y_set = y_set;
else
    %此if分支表示不是首次运行
    %对每个x_set上的点做处理
    for i = 1 : length(x_set)
        %不是首次运行，对于点x_set(i),y_set(i)来说,start_search_index =
        %pre_match_point_index_set(i)
        start_search_index = pre_match_point_index_set(i);%上个周期匹配点的编号作为本周期搜索的起点
        % 判断帧与帧之间的障碍物是否为同一个
        square_dis = (x_set(i) - pre_x_set(i))^2 + (y_set(i) - pre_y_set(i))^2;
        if square_dis > 36
            % 帧与帧之间的物体的位置距离过大，认为是两个障碍物
            start_search_index = nan;
        end
        % 声明increase_count，用于表示在遍历时distance连续增加的个数
        %%%%%%%%%
        %对于障碍物检测而言，当感知第一次检测到障碍物时，算法并不是首次运行，此时 
        %pre_match_point_index_set的值是nan，如果还用上一时刻的结果作为本周期搜索的起点
        %必然会出问题，所以要修改
        % 声明increase_count_limit
        increase_count_limit = 5;
        if isnan(start_search_index)
            %没有上个周期的结果，那就不能只检查5次了
            increase_count_limit = 50;
            %搜索起点也要设为1
            start_search_index = 1;
        end
        increase_count = 0;
        % 开始遍历
        %这里多一个步骤，判断遍历的方向
        %计算上个周期匹配点的位矢
        vector_pre_match_point = [pre_frenet_path_x(start_search_index);pre_frenet_path_y(start_search_index)];
        vector_pre_match_point_direction = ...
            [cos(pre_frenet_path_heading(start_search_index));sin(pre_frenet_path_heading(start_search_index))];
        %判断遍历的方向
        flag = ([x_set(i);y_set(i)] - vector_pre_match_point)' * vector_pre_match_point_direction;
        min_distance = inf;
        if flag > 0.001
            for j = start_search_index : length(frenet_path_x)
                distance = (x_set(i) - frenet_path_x(j))^2 + (y_set(i) - frenet_path_y(j))^2;
                if distance < min_distance
                    min_distance = distance;
                    match_point_index_set(i) = j;
                    increase_count = 0;
                else
                    increase_count = increase_count + 1;
                end
                %如果distance连续增加increase_count_limit次就不要再遍历了，节省时间
                if increase_count > increase_count_limit
                    break;
                end
            end
        elseif flag < - 0.001
            for j = start_search_index : -1 : 1
                distance = (x_set(i) - frenet_path_x(j))^2 + (y_set(i) - frenet_path_y(j))^2;
                if distance < min_distance
                    min_distance = distance;
                    match_point_index_set(i) = j;
                    increase_count = 0;
                else
                    increase_count = increase_count + 1;
                end
                %如果distance连续增加increase_count_limit次就不要再遍历了，节省时间
                if increase_count > increase_count_limit
                    break;
                end
            end
        else
            match_point_index_set(i) = start_search_index;
        end
        
        %如何通过匹配点计算投影点，请参见《自动驾驶控制算法第七讲》
        %或《自动驾驶决策规划算法》第一章第三节
        
        %取出匹配点的编号
        match_point_index = match_point_index_set(i);
        %取出匹配点的信息
        match_point_x = frenet_path_x(match_point_index);
        match_point_y = frenet_path_y(match_point_index);
        match_point_heading = frenet_path_heading(match_point_index);
        match_point_kappa = frenet_path_kappa(match_point_index);
        %计算匹配点的方向向量与法向量
        vector_match_point = [match_point_x;match_point_y];
        vector_match_point_direction = [cos(match_point_heading);sin(match_point_heading)];
        %声明待投影点的位矢
        vector_r = [x_set(i);y_set(i)];
        
       %通过匹配点计算投影点
       vector_d = vector_r - vector_match_point;
       ds = vector_d' * vector_match_point_direction;
       vector_proj_point = vector_match_point + ds * vector_match_point_direction;
       proj_heading = match_point_heading + match_point_kappa * ds;
       proj_kappa = match_point_kappa;
       %计算结果输出
       proj_x_set(i) = vector_proj_point(1);
       proj_y_set(i) = vector_proj_point(2);
       proj_heading_set(i) = proj_heading;
       proj_kappa_set(i) = proj_kappa;
  
    end
    %匹配点的计算结果保存，供下一个周期使用
    pre_match_point_index_set = match_point_index_set;
    pre_frenet_path_x = frenet_path_x;
    pre_frenet_path_y = frenet_path_y;
    pre_frenet_path_heading = frenet_path_heading;
    pre_frenet_path_kappa = frenet_path_kappa;
    pre_x_set = x_set;
    pre_y_set = y_set;
end

== matlab function planner_contral/decision_planning/referenceline provider/calculate heading&kappa ==
  data: path_x input; path_heading output; path_y input; path_kappa output
function [path_heading,path_kappa] = fcn(path_x,path_y)
%该函数将计算path的切线方向与x轴的夹角和曲率
%输入：path_x,y路径坐标
%输出：path heading kappa 路径的heading和曲率
%原理 heading = arctan(dy/dx);
%     kappa = dheading/ds;
%     ds = (dx^2 + dy^2)^0.5

%注意，角度的多值性会带来很大的麻烦，需要慎重处理
%例，x 与 x + 2pi往往代表同一个角度，这种多值性在计算曲率会带来麻烦
%比如 原本是(0.1 - (-0.1))/ds，但如果计算出的-0.1多了一个2pi
%kappa就等于(0.1 - (-0.1 + 2*pi))/ds，曲率会变得非常大
%还有若采用中点欧拉法计算heading时，(即使用(y2 - y1)/(x2 - x1)的反正切计算一个角度 ，用(y1 - y0)/(x1
%-x0)的反正切又计算一个角度，然后加起来除以2),如果精确值是 (a1 + a2)/2,但最终计算的结果可能是(a1 + a2 + 2pi)/2
% 还有 tan(x) = tan(x + pi) 所以arctan(tan(x))可能等于x，也可能等于x + pi
% 角度的处理非常麻烦，而且角度处理不当往往是许多奇怪错误的源头

dx = diff(path_x);
dy = diff(path_y);
%用中点欧拉法要比向前欧拉法向后欧拉法更精确，但是也可能计算出的结果比精确值多一个pi
%在这里对dx,dy做中点欧拉法，使用四象限反正切计算角度
dx_pre = [dx(1);dx];
dx_after = [dx;dx(end)];
dx_final = (dx_pre + dx_after)/2;

dy_pre = [dy(1);dy];
dy_after = [dy;dy(end)];
dy_final = (dy_pre + dy_after)/2;

ds_final = sqrt(dx_final.^2 + dy_final.^2);
path_heading = atan2(dy_final,dx_final);

dheading = diff(path_heading);
dheading_pre = [dheading(1);dheading];
dheading_after = [dheading;dheading(end)];
dheading_final = (dheading_pre + dheading_after) / 2;
%为了防止dheading出现多一个2pi的错误，假设真实的dheading较小，用sin(dheading)近似dheading
path_kappa = sin(dheading_final) ./ ds_final;

== matlab function planner_contral/decision_planning/EMplanner/calc speed planning start condition ==
  data: plan_start_vx input; plan_start_s_dot output; plan_start_vy input; plan_start_ax input; plan_start_ay input; plan_start_heading input; plan_start_s_dot2 output
function [plan_start_s_dot,plan_start_s_dot2] = fcn(plan_start_vx,plan_start_vy,plan_start_ax,plan_start_ay,plan_start_heading)
% 该函数计算速度规划的初始条件
tor = [cos(plan_start_heading);sin(plan_start_heading)];
v_t = tor'*[plan_start_vx;plan_start_vy];
a_t = tor'*[plan_start_ax;plan_start_ay];
plan_start_s_dot = v_t;
plan_start_s_dot2 = a_t;
